simulink model "F16_longitudinal_nonlinear_simulation_R2018a"  (R2018a)
settings: Solver=VariableStepAuto  StartTime=0.0  StopTime=60  MaxStep=1.2  RelTol=1e-3
libraries: simulink x3, aerolibanimutils x1
settings Model: Creator=parth  LastModifiedBy=parth
settings DataIOCC: ReturnWorkspaceOutputs=on
settings SFSimCC: SimUseLocalCustomCode=on
settings RTWCC: RTWUseLocalCustomCode=on

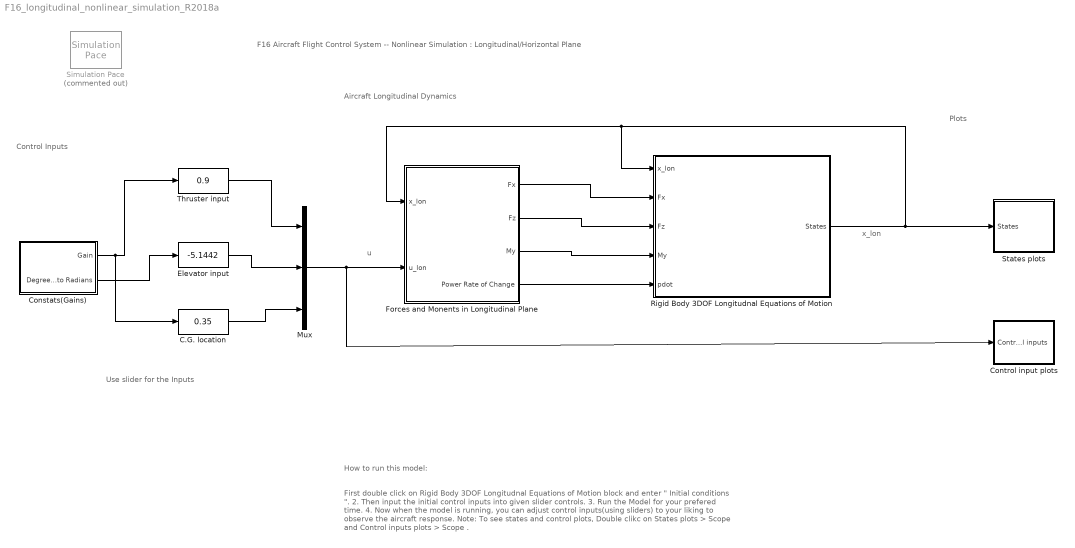
== system F16_longitudinal_nonlinear_simulation_R2018a ==
  note: u
  note: x_lon
  note: Plots
  note: Use slider for the Inputs
  note: F16 Aircraft Flight Control System -- Nonlinear Simulation : Longitudinal/Horizontal Plane
  note: Control Inputs
  note: Aircraft Longitudinal Dynamics
  note: First double click on Rigid Body 3DOF Longitudnal Equations of Motion block and enter " Initial conditions ".
      | 2. Then input the initial control inputs into given slider controls.
      | 3. Run the Model for your prefered time.
      | 4. Now when the model is running, you can adjust control inputs(using sliders) to your liking to observe the aircraft response.
      |
      | Note: To see states and control plots, Double clikc on States plots > Scope and Control inputs plots > Scope .
  note: How to run this model:
  C.G. location : simulink/Math Operations/Slider Gain  gain=0.35  low=0.3  high=0.4
  Constats(Gains) : Subsystem
  Control input plots : Subsystem
  Elevator input : simulink/Math Operations/Slider Gain  gain=-5.1442  low=-25  high=25
  Forces and Monents in Longitudinal Plane : Subsystem
  Mux : Mux  Inputs=3
  "Rigid Body 3DOF Longitudnal Equations of Motion " : Subsystem  mask{V_init=500, alpha_init=-0.16395, q_init=0.3, theta_init=-0.16395, Xe_init=0, h_init=0, actual_power_init=57.3271}
      mask prompts: V_init "V_init (ft/sec)"; alpha_init "alpha_init (rad)"; q_init "q_init (rad/sec)"; theta_init "theta_init (rad)"; Xe_init "Xe_init (ft)"; h_init "h_init (ft)"
      mask DialogControl ParameterGroupVar Prompt: Enter Aircraft Initial States here:
  Simulation Pace : aerolibanimutils/Simulation Pace  Commented=on  SimulationPace=1  SleepMode=Auto  OutputPaceError=off  SampleTime=1/30
  States plots : Subsystem
  Thruster input : simulink/Math Operations/Slider Gain  gain=0.9  low=0  high=1
  wires:
  Mux/1 -> Control input plots/1(Control inputs), Forces and Monents in Longitudinal Plane/2(u_lon)
  Thruster input/1 -> Mux/1
  Elevator input/1 -> Mux/2
  Forces and Monents in Longitudinal Plane/4(Power Rate of Change) -> "Rigid Body 3DOF Longitudnal Equations of Motion "/5(pdot)
  Constats(Gains)/1(" Gain") -> C.G. location/1, Thruster input/1
  Forces and Monents in Longitudinal Plane/1(Fx) -> "Rigid Body 3DOF Longitudnal Equations of Motion "/2(Fx)
  Forces and Monents in Longitudinal Plane/2(Fz) -> "Rigid Body 3DOF Longitudnal Equations of Motion "/3(Fz)
  Constats(Gains)/2(Degree to Radians) -> Elevator input/1
  "Rigid Body 3DOF Longitudnal Equations of Motion "/1(States) -> Forces and Monents in Longitudinal Plane/1(x_lon), "Rigid Body 3DOF Longitudnal Equations of Motion "/1(x_lon), States plots/1(States)
  Forces and Monents in Longitudinal Plane/3(My) -> "Rigid Body 3DOF Longitudnal Equations of Motion "/4(My)
  C.G. location/1 -> Mux/3

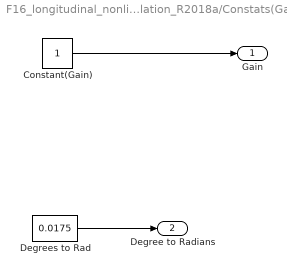
== system F16_longitudinal_nonlinear_simulation_R2018a/Constats(Gains) ==
  Constant(Gain) : Constant
  Degrees to Rad : Constant  Value=0.0175
  " Gain" : Outport
  Degree to Radians : Outport  Port=2
  wires:
  Degrees to Rad/1 -> Degree to Radians/1
  Constant(Gain)/1 -> " Gain"/1

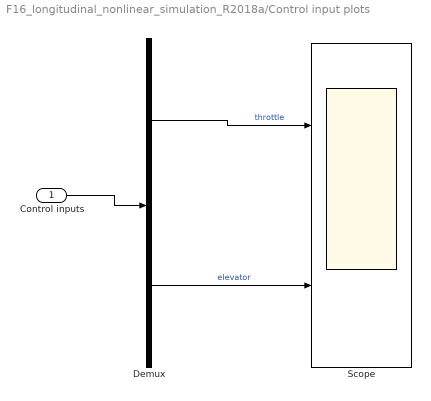
== system F16_longitudinal_nonlinear_simulation_R2018a/Control input plots ==
  Control inputs : Inport
  Demux : Demux  Outputs=2
  Scope : Scope  NumInputPorts=2
  wires:
  Demux/1 -> Scope/1  "throttle"
  Control inputs/1 -> Demux/1
  Demux/2 -> Scope/2  "elevator"

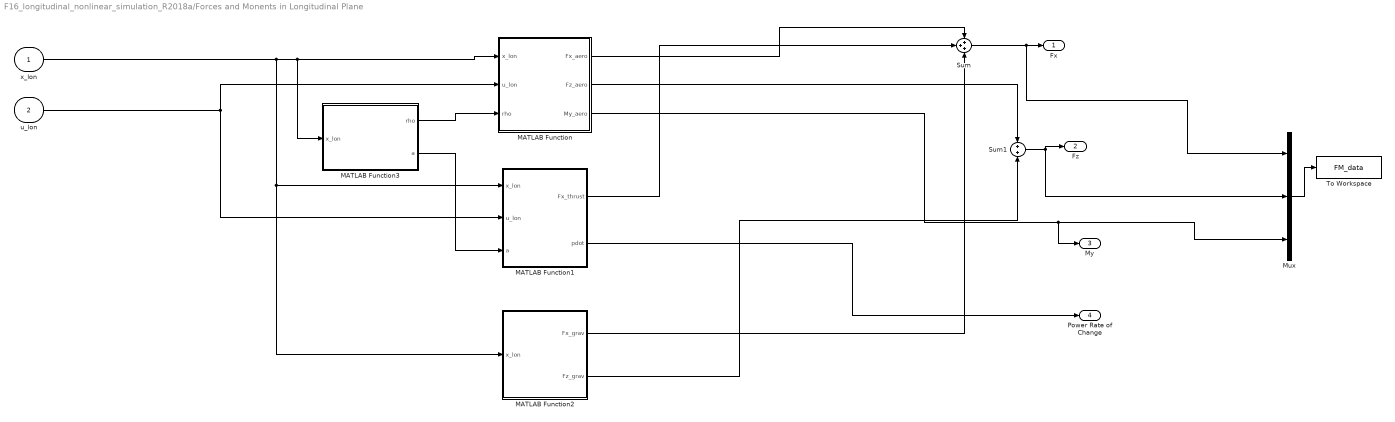
== system F16_longitudinal_nonlinear_simulation_R2018a/Forces and Monents in Longitudinal Plane ==
  x_lon : Inport
  u_lon : Inport  Port=2
  MATLAB Function : MATLAB Function  TreatAsAtomicUnit=on
  MATLAB Function1 : MATLAB Function  TreatAsAtomicUnit=on
  MATLAB Function2 : MATLAB Function  TreatAsAtomicUnit=on
  MATLAB Function3 : MATLAB Function  TreatAsAtomicUnit=on
  Mux : Mux  Inputs=3
  Sum : Sum  Inputs=+++
  Sum1 : Sum
  To Workspace : ToWorkspace  VariableName=FM_data  SaveFormat=Timeseries  SampleTime=-1
  Fx : Outport
  Fz : Outport  Port=2
  My : Outport  Port=3
  Power Rate of Change : Outport  Port=4
  wires:
  x_lon/1 -> MATLAB Function2/1(x_lon), MATLAB Function1/1(x_lon), MATLAB Function3/1(x_lon), MATLAB Function/1(x_lon)
  u_lon/1 -> MATLAB Function1/2(u_lon), MATLAB Function/2(u_lon)
  MATLAB Function1/2(pdot) -> Power Rate of Change/1
  MATLAB Function3/1(rho) -> MATLAB Function/3(rho)
  MATLAB Function3/2(a) -> MATLAB Function1/3(a)
  MATLAB Function/1(Fx_aero) -> Sum/1
  MATLAB Function1/1(Fx_thrust) -> Sum/2
  MATLAB Function2/1(Fx_grav) -> Sum/3
  Sum/1 -> Mux/1, Fx/1
  MATLAB Function/2(Fz_aero) -> Sum1/1
  Sum1/1 -> Mux/2, Fz/1
  MATLAB Function2/2(Fz_grav) -> Sum1/2
  MATLAB Function/3(My_aero) -> Mux/3, My/1
  ? -> ?
  Mux/1 -> To Workspace/1

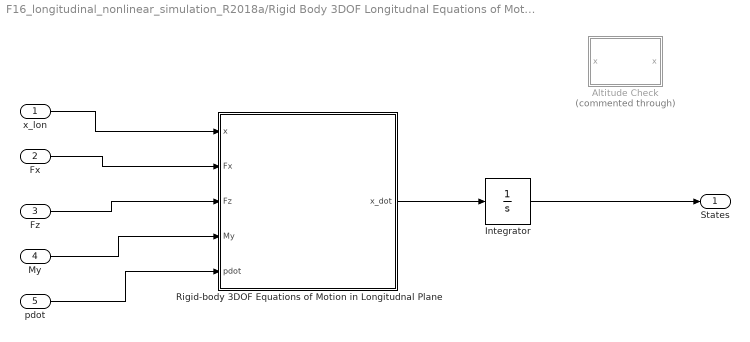
== system F16_longitudinal_nonlinear_simulation_R2018a/Rigid Body 3DOF Longitudnal Equations of Motion  ==
  x_lon : Inport
  Fx : Inport  Port=2
  Fz : Inport  Port=3
  My : Inport  Port=4
  pdot : Inport  Port=5
  Altitude Check : MATLAB Function  Commented=through  TreatAsAtomicUnit=on
  Integrator : Integrator  InitialCondition=[(V_init*cos(alpha_init)); (V_init*sin(alpha_init)); q_init; theta_init; Xe_init; h_init; actual_power_init]
  Rigid-body 3DOF Equations of Motion in Longitudnal Plane : MATLAB Function  TreatAsAtomicUnit=on
  States : Outport
  wires:
  Fx/1 -> Rigid-body 3DOF Equations of Motion in Longitudnal Plane/2(Fx)
  x_lon/1 -> Rigid-body 3DOF Equations of Motion in Longitudnal Plane/1(x)
  Rigid-body 3DOF Equations of Motion in Longitudnal Plane/1(x_dot) -> Integrator/1
  pdot/1 -> Rigid-body 3DOF Equations of Motion in Longitudnal Plane/5(pdot)
  Fz/1 -> Rigid-body 3DOF Equations of Motion in Longitudnal Plane/3(Fz)
  Integrator/1 -> States/1
  My/1 -> Rigid-body 3DOF Equations of Motion in Longitudnal Plane/4(My)

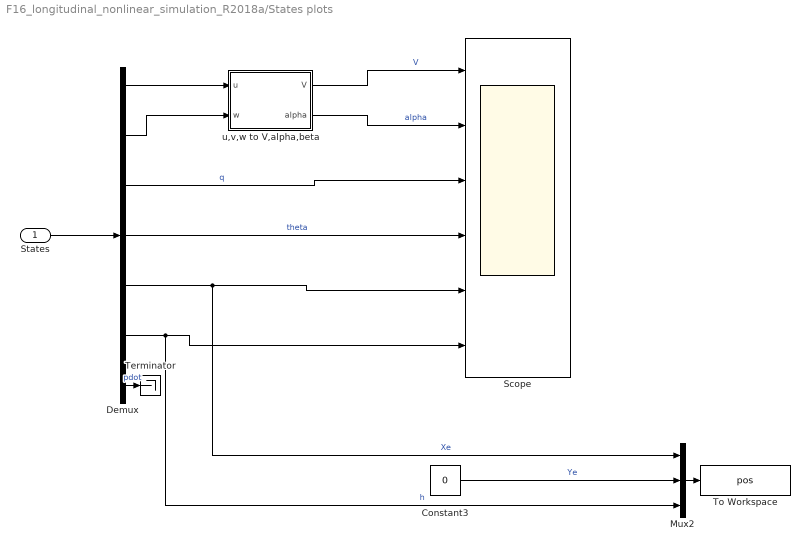
== system F16_longitudinal_nonlinear_simulation_R2018a/States plots ==
  States : Inport
  Constant3 : Constant  Value=0
  Demux : Demux  Outputs=7
  Mux2 : Mux  Inputs=3
  Scope : Scope  NumInputPorts=6
  Terminator : Terminator
  To Workspace : ToWorkspace  VariableName=pos  SaveFormat=Timeseries  SampleTime=-1
  u,v,w to V,alpha,beta : MATLAB Function  TreatAsAtomicUnit=on
  wires:
  Demux/1 -> u,v,w to V,alpha,beta/1(u)
  Demux/2 -> u,v,w to V,alpha,beta/2(w)
  Demux/3 -> Scope/3  "q"
  States/1 -> Demux/1
  u,v,w to V,alpha,beta/2(alpha) -> Scope/2  "alpha"
  u,v,w to V,alpha,beta/1(V) -> Scope/1  "V"
  Demux/7 -> Terminator/1  "pdot"
  Demux/4 -> Scope/4  "theta"
  Mux2/1 -> To Workspace/1
  Constant3/1 -> Mux2/2  "Ye"
  Demux/6 -> Mux2/3, Scope/6  "h"
  Demux/5 -> Mux2/1, Scope/5  "Xe"

== matlab function F16_longitudinal_nonlinear_simulation_R2018a/Forces and Monents in Longitudinal Plane/MATLAB Function1 ==
  data: x_lon input; Fx_thrust output; u_lon input; pdot output; a input
function [Fx_thrust, pdot] = F16_propulsion(x_lon,u_lon,a)
%Calculate Propulsive Forces and Moments 
% u_lon = [delta_T, delta_e]
%
% based on work for Stanle Bak
% https://github.com/stanleybak/AeroBenchVVPython

%% TGEAR function
% convert command [0,1] to commanded power [0,100]
if (u_lon(1) <= .77)
    comm_power = 64.94 * u_lon(1);  % commanded power
else
    comm_power = 217.38 * u_lon(1) - 117.38;
end

%% RTAU function
% time constant for first order lag in engine power dynamic repsonse
    function rt = rtau(delta_power)
        if(delta_power <= 25)
            rt = 1.0;
        elseif(delta_power >= 50)
            rt = .1;
        else
            rt = 1.9 - .036*delta_power;
        end
    end
    
%% PDOT function
% comptute rate of change power fromm given actual power and commanded
% power
if(comm_power >= 50)
    if(x_lon(7) >= 50)
        t = 5;
        p2 = comm_power;
    else
        p2 = 60;
        t = rtau(p2 - x_lon(7));
    end
else
    if (x_lon(7) >= 50)
        t = 5;
        p2 = 40;
    else
        p2 = comm_power;
        t = rtau(p2 - x_lon(7));
    end
end

pdot = t * (p2 - x_lon(7));

%% THRUST function
% calculate engine thrust
V = sqrt(x_lon(1)^2 + x_lon(2)^2);
M = V/a; % mach number

a = [1060,670,880,1140,1500,1860;...
    635,425,690,1010,1330,1700;...
    60,25,345,755,1130,1525;...
    -1020,-170,-300,350,910,1360;...
    -2700,-1900,-1300,-247,600,1100;...
    -3600,-1400,-595,-342,-200,700]';

b = [12680,9150,6200,3950,2450,1400;...
    12680,9150,6313,4040,2470,1400;...
    12610,9312,6610,4290,2600,1560;...
    12640,9839,7090,4660,2840,1660;...
    12390,10176,7750,5320,3250,1930;...
    11680,9848,8050,6100,3800,2310;]';

c = [20000,15000,10800,7000,4000,2500;...
    21420,15700,11225,7323,4435,2600;...
    22700,16860,12250,8154,5000,2835;...
    24240,18910,13760,9285,5700,3215;...
    26070,21075,15975,11115,6860,3950;...
    28886,23319,18300,13484,8642,5057]';

if (x_lon(6)<0)
    x_lon(6) = 0.01;
end

h =.0001 * x_lon(6);
i = fix(h);  
if(i >= 5)
    i = 4;
end

dh = h - i;
rm = 5 * M;
m = fix(rm);
if(m >= 5)
    m = 4;
end

dm = rm - m;
cdh = 1 - dh;

i = i + 1;
m = m + 1;

s = b(i, m) * cdh + b(i + 1, m) * dh;
t = b(i, m + 1) * cdh + b(i + 1, m + 1) * dh;
tmil = s + (t - s) * dm;

% Fx_thrust == thrust
if (x_lon(7) < 50)
    s = a(i, m) * cdh + a(i + 1, m) * dh;
    t = a(i, m + 1) * cdh + a(i + 1, m + 1) * dh;
    tidl = s + (t - s) * dm;
    Fx_thrust = tidl + (tmil - tidl) * x_lon(7) * .02;
else 
    s = c(i, m) * cdh + c(i + 1, m) * dh;
    t = c(i, m + 1) * cdh + c(i + 1, m + 1) * dh;
    tmax = s + (t - s) * dm;
    Fx_thrust = tmil + (tmax - tmil) * (x_lon(7) - 50) * .02;
end

end

== matlab function F16_longitudinal_nonlinear_simulation_R2018a/Forces and Monents in Longitudinal Plane/MATLAB Function ==
  data: x_lon input; Fx_aero output; u_lon input; Fz_aero output; rho input; My_aero output
function [Fx_aero, Fz_aero,My_aero] = F16_aerodynamics(x_lon,u_lon,rho)
% Compute F16 Body-axis Aerodynamics forces and moments
% u_lon = [delta_T, delta_e]
%
% Arodynamic model for F16 in form of Polynomial function
% is used here instead of data tables as described in [1]
%
% Ref:
% [1] GLOBAL NONLINEAR PARAMETRIC MODELING WITH APPLICATION TO 
%     F-16 AERODYNAMICS, by Eugene A. Morelli.

% physical parameters
% Ref: Aircraft Control and Simulation, Stevens & Lewis.
S = 300; % wing area, ft^2
c_bar = 11.32; % mean aero cord, ft
b = 30; % wing span, ft
xcg_ref = 0.35;%*c_bar; % reference c.g. location
x_cg = u_lon(3);%*c_bar; % c.g. location % VARIABLE % Fixed here

% convert body-axis velocity to (alpha,beta,V)
V = sqrt(x_lon(1)^2 + x_lon(2)^2); % m/sec
alpha = atan(x_lon(2)/x_lon(1)); % rad

% variable ranges  % bound
%    -- Table 1 [1]
if alpha < -0.1745      % -10 to 45 deg
    alpha = -0.1745;
elseif alpha > 0.7854
    alpha = 0.7854;
end
beta = 0; % for longitudinal plane motion

% aerodynamic polynomial model
%    -- Table 2 [1]
Cx_0 = -1.943367e-02 + 2.136104e-01*alpha - 2.903457e-01*(u_lon(2)^2) ...
       -3.348641e-03*u_lon(2) - 2.060504e-01*alpha*u_lon(2) + ...
       6.988016e-01*(alpha^2) - 9.035381e-01*(alpha^3);
Cx_q = 4.833383e-01 + 8.644627e+00*alpha + 1.131098e+01*(alpha^2) ...
       - 7.422961e+01*(alpha^3) + 6.075776e+01*(alpha^4);
Cz_0 = (1-(beta^2))*(-1.378278e-01 - 4.211369e+00*alpha + ...
        4.775187e+00*(alpha^2) - 1.026225e+01*(alpha^3) + ...
        8.399763e+00*(alpha^4)) - 4.354000e-01*u_lon(2);
Cz_q = -3.054956e+01 - 4.132305e+01*alpha + 3.292788e+02*(alpha^2) ...
       - 6.848038e+02*(alpha^3) + 4.080244e+02*(alpha^4);
Cm_0 = -2.029370e-02 + 4.660702e-02*alpha - 6.012308e-01*u_lon(2) ...
       -8.062977e-02*alpha*u_lon(2) + 8.320429e-02*(u_lon(2)^2) + ...
       5.018538e-01*(alpha^2)*u_lon(2) + 6.378864e-01*(u_lon(2)^3) ...
       + 4.226356e-01*alpha*(u_lon(2)^2);
Cm_q = -5.159153e+00 - 3.554716e+00*alpha - 3.598636e+01*(alpha^2) + ...
       2.247355e+02*(alpha^3) - 4.120991e+02*(alpha^4) ...
       + 2.411750e+02*(alpha^5);
   
% dynamic pressure
q_bar = 0.5*rho*V*V;

% non-dimensional
q_nd = 0.5*x_lon(3)*c_bar/V;

% aerodynamic forces
Cx = Cx_0 + q_nd*Cx_q;
Cz = Cz_0 + q_nd*Cz_q;

% aerodynamic moments
Cm = Cm_0 + q_nd*Cm_q + Cz*(xcg_ref - x_cg);

Fx_aero = q_bar*S*Cx;
Fz_aero = q_bar*S*Cz;
My_aero = q_bar*S*Cm*c_bar;
end

== matlab function F16_longitudinal_nonlinear_simulation_R2018a/Forces and Monents in Longitudinal Plane/MATLAB Function2 ==
  data: x_lon input; Fx_grav output; Fz_grav output
function [Fx_grav, Fz_grav] = gravity_model(x_lon)
% Gravity forces and moments in body axis system
% 
% References : Ch. 7, Aircraft Flight Dynamics and Control,
%               by Wayne Durham.

g = 32.17; %ft/s^2
Fx_grav = -g*sin(x_lon(4));
Fz_grav = g*cos(x_lon(4));
end

== matlab function F16_longitudinal_nonlinear_simulation_R2018a/Rigid Body 3DOF Longitudnal Equations of Motion /Rigid-body 3DOF Equations of Motion in Longitudnal Plane ==
  data: x input; x_dot output; Fx input; Fz input; My input; pdot input
function x_dot = nonlinear_3DOF_longitudinal(x, Fx, Fz, My, pdot)
% rigid body aircraft 3DOF nonlinear equations of motion
% in Longtudinal Plane,
% in Body-axis with Flat Earth Assumption.
% x = [u,w,q,theta,xe,h(=ze)), pdot]  ==> must be (7,1)
%%%% u = [delta_T, delta_e]

%%%% delta_T -> between 0 to 1
%%%% delta_e, delta_a, delta_r -> rad

% References : INTRODUCTION TO AIRCRAFT FLIGHT MECHANICS
%               by Yechout et all. Page no. 164

% physical parameters
% Ref: Aircraft Control and Simulation, Stevens & Lewis.
m = 637.2397; %20500/32.17; % lbs

Iyy = 55814;

%% Equations of Motion (Body axis)
x_dot = zeros(7,1);
x_dot(1,1) = (Fx/m) - x(3)*x(2); % udot
x_dot(2,1) = (Fz/m) + x(3)*x(1); % wdot
x_dot(3,1) = My/Iyy; % qdot
x_dot(4,1) = x(3); % thetadot
x_dot(5,1) = x(1)*cos(x(4)) + x(2)*sin(x(4)); % Xedot
x_dot(6,1) = x(1)*sin(x(4)) - x(2)*cos(x(4)); %hdot
x_dot(7,1) = pdot; % pdot
end

== matlab function F16_longitudinal_nonlinear_simulation_R2018a/Forces and Monents in Longitudinal Plane/MATLAB Function3 ==
  data: x_lon input; rho output; a output
function [rho, a] = atmospheric_model(x_lon)
% calculate the atmospheric density(in Kg/m^3) and speed of sound
% at the given altitude
% 
% Ref: Stevens & Lewis, "Aircraft Control and Simulation"

    altitude = x_lon(6);
    ro = 2.377e-3;
    tfac = 1 - .703e-5 * altitude;

    if altitude >= 35000 % in stratosphere
        t = 390;
    else
        t = 519 * tfac; % 3 rankine per atmosphere (3 rankine per 1000 ft)
    end
    rho = ro * tfac^4.14;

    %speed of sound
    a = sqrt(1.4 * 1716.3 * t);

end

== matlab function F16_longitudinal_nonlinear_simulation_R2018a/Rigid Body 3DOF Longitudnal Equations of Motion /Altitude Check ==
  data: x input; x output
function x = fcn(x)

% Altitude check
if (x(6) <= 0.01)
    x(6) = 0.01;
end

end

== matlab function F16_longitudinal_nonlinear_simulation_R2018a/States plots/u,v,w to V,alpha,beta ==
  data: u input; V output; w input; alpha output
function [V,alpha] = fcn(u,w)

V = sqrt(u^2 + w^2);
alpha = atan(w/u);
end
